simulink model "exp80x5B10x5D1"  (R2024a)
settings: Solver=FixedStepAuto  StartTime=0.0  StopTime=1  FixedStep=25e-6  RelTol=1e-3
undefined symbols (not defined in the file): Ion, Lithium
libraries: spsDiodeLib x4, spsSeriesRLCBranchLib x3, spsIGBTDiodeLib x2, spsACVoltageSourceLib x1, spsBatteryLib x1, spsLinearTransformerLib x1, spsVoltageMeasurementLib x1, sps_lib x1
settings Model: Creator=archi  LastModifiedBy=kumar
settings RTWCC: GPUComputeCapability=3.5

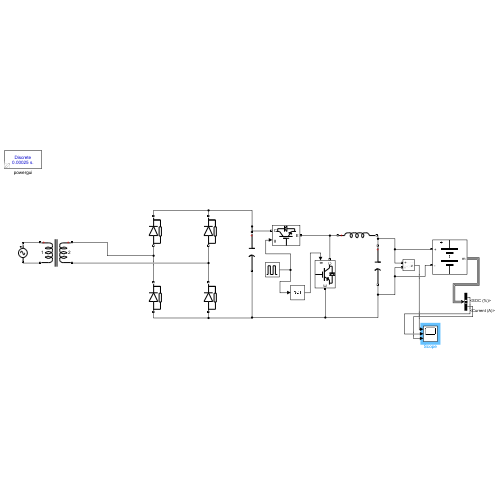
[thumbnail: Simulink's stored preview of the top-level diagram]
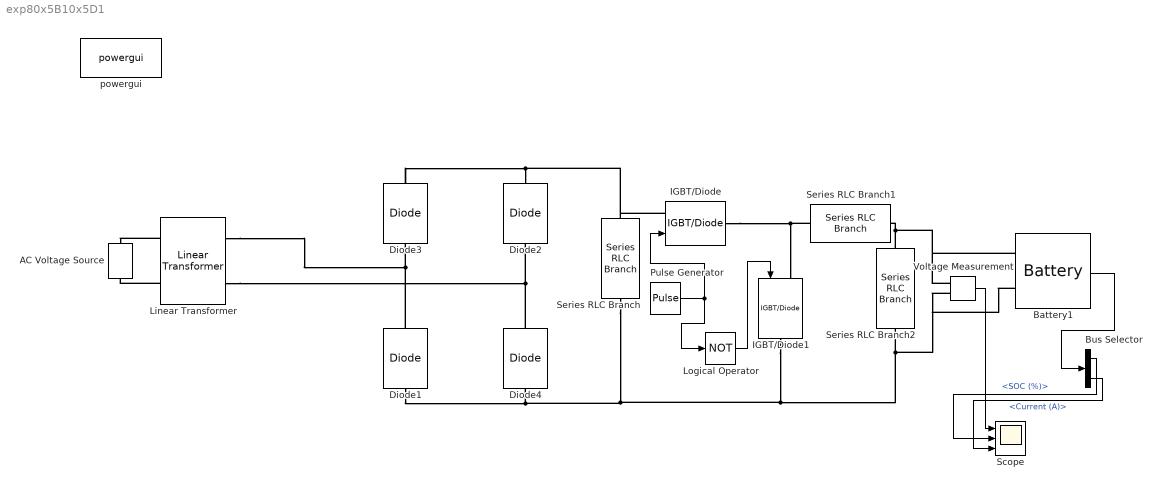
== system exp80x5B10x5D1 ==
  AC Voltage Source : spsACVoltageSourceLib/AC Voltage Source  Amplitude=230*sqrt(2)  Phase=0  Frequency=50  SampleTime=0  Measurements=None  BusType=swing  Pref=10e3  Qref=0  Qmin=-inf  Qmax=+inf
  Battery1 : spsBatteryLib/Battery  BatType=Lithium-Ion  ShowTempParam=off  ThermalPreset=no  ShowAgeParam=off  NomV=12  NomQ=18  SOC=50  Batt_Tr=30  PresetModel=on  MaxQ=18  MinV=9  FullV=13.9678  Dis_rate=7.8261  R=0.0066667  Normal_OP=16.2783  expZone="[12.9646     0.884348]"  current=[6.5 13 32.5]  Units=Time  Tci=20  NomT=20  T2=-30  MaxQ2=4.8  FullV2=7.1  Normal_OP2=5.655  expZone2="[6.58           1]"  Rca=0.6  ti=2000  Dp=0  Neq0=0  Tsim=1e6  Ta1=25  Qeol=5.4*0.9  Reol=0.013333*1.2  Char_age=[2.3478, 3]  Dis_age=[2.3478, 10]  N1=1500  N2=10500  N3=1000  N4=1400  Ta2=45  N5=950
  Bus Selector : BusSelector  OutputSignals=SOC (%),Current (A)
  Diode{1..4} (4 alike) : spsDiodeLib/Diode  Ron=0.001  Lon=0  Vf=0.8  IC=0  UseSnubber=0  Rs=500  Cs=250e-9  Measurements=off
  IGBT/Diode : spsIGBTDiodeLib/IGBT//Diode  Ron=1e-3  Rs=1e5  Cs=inf  Measurements=off
  IGBT/Diode1 : spsIGBTDiodeLib/IGBT//Diode  Ron=1e-3  Rs=1e5  Cs=inf  Measurements=off
  Linear Transformer : spsLinearTransformerLib/Linear Transformer  UNITS=pu  NominalPower=[500 50 ]  winding1="[ 230  0.002  0.08 ]"  winding2="[ 24  0.002  0.08 ]"  ThreeWindings=off  winding3=[ 315e3 0.002 0.08 ]  RmLm=[ 500 500 ]  Measurements=None  DataType=off
  Logical Operator : Logic  Operator=NOT  AllPortsSameDT=off  OutDataTypeStr=boolean
  Pulse Generator : DiscretePulseGenerator  PulseType=Time based  Period=1/5000  PulseWidth=50
  Scope : Scope  NumInputPorts=3
  Series RLC Branch : spsSeriesRLCBranchLib/Series RLC Branch  LConnTagsString=__new0  RConnTagsString=__new0  BranchType=C  Resistance=1  Inductance=1e-3  SetiL0=off  InitialCurrent=0  Capacitance=1000e-6  Setx0=off  InitialVoltage=0  Measurements=None
  Series RLC Branch1 : spsSeriesRLCBranchLib/Series RLC Branch  LConnTagsString=__new0  RConnTagsString=__new0  BranchType=L  Resistance=1  Inductance=50e-3  SetiL0=off  InitialCurrent=0  Capacitance=1e-6  Setx0=off  InitialVoltage=0  Measurements=None
  Series RLC Branch2 : spsSeriesRLCBranchLib/Series RLC Branch  LConnTagsString=__new0  RConnTagsString=__new0  BranchType=C  Resistance=1  Inductance=1e-3  SetiL0=off  InitialCurrent=0  Capacitance=25e-6  Setx0=off  InitialVoltage=0  Measurements=None
  Voltage Measurement : spsVoltageMeasurementLib/Voltage Measurement  PhasorSimulation=off  OutputType=Complex  PSBequivalent=0
  powergui : sps_lib/powergui  Priority=1  SimulationMode=Discrete  SampleTime=25e-5  frequency=60  Iterations=50  frequencyindice=0  Pbase=100e6  ErrMax=1e-4  UnitsV=kV  UnitsW=MW  buscounter=0  FunctionMessages=off  echomessages=off  EnableUseOfTLC=off  CurrentSourceSwitches=off  DisableSnubberDevices=off  DisableRonSwitches=off  DisableVfSwitches=off  DisplayEquations=off  AutomaticDiscreteSolvers=off  SolverType=Tustin/Backward Euler (TBE)  Interpol=off  ExternalGateDelay=off  methode=off  Ts=100  x0status=blocks  SPID=on  SwTol=0  HookPort=off  NonlinearTolerance=1e-4  nMaxIteration=100  ContinueOnMaxIteration=off  RestoreLinks=warning  ResistiveCurrentMeasurement=off  Frange=[0:2:500]  Ylog=off  Xlog=on  ShowGrid=off  save=off  variable=ZData  structure=0  ZoomFFT=off  StartTime=0.0  cycles=1  DisplayStyle=1  fundamental=60  FreqAxis=off  MaxFrequency=1000  frequencyindicesteady=1  RmsSteady=1  display=off
  wires:
  Pulse Generator/1 -> Logical Operator/1, IGBT/Diode/1
  Logical Operator/1 -> IGBT/Diode1/1
  Voltage Measurement/1 -> Scope/1
  Battery1/1 -> Bus Selector/1
  Bus Selector/1 -> Scope/2  "<SOC (%)>"
  Bus Selector/2 -> Scope/3  "<Current (A)>"
  connections:
  IGBT/Diode/RConn1 -- Series RLC Branch1/LConn1 -- IGBT/Diode1/LConn1
  Series RLC Branch2/LConn1 -- Battery1/LConn1 -- Voltage Measurement/LConn1 -- Series RLC Branch1/RConn1
  Diode4/RConn1 -- Linear Transformer/RConn2 -- Diode2/LConn1
  Diode1/RConn1 -- Linear Transformer/RConn1 -- Diode3/LConn1
  Diode3/RConn1 -- IGBT/Diode/LConn1 -- Series RLC Branch/LConn1 -- Diode2/RConn1
  IGBT/Diode1/RConn1 -- Battery1/LConn2 -- Voltage Measurement/LConn2 -- Series RLC Branch2/RConn1 -- Diode1/LConn1 -- Diode4/LConn1 -- Series RLC Branch/RConn1
  Linear Transformer/LConn1 -- AC Voltage Source/RConn1
  Linear Transformer/LConn2 -- AC Voltage Source/LConn1
